simulink model "tanks_3_mathworks"  (Simulink 8.7)
settings: Solver=VariableStepAuto  StartTime=0.0  StopTime=700.0  RelTol=1e-3
values from neighbouring files (symbols this model uses):
  A1 = 4.9    [defineProcess_basic_outputs.m]
  g = 981    [defineProcess_basic_outputs.m]
  g1 = 0.3    [defineProcess_basic_outputs.m]
  g2 = 0.3    [defineProcess_basic_outputs.m]
  h1 = 10    [defineProcess_basic_outputs.m]
  h2 = 10    [defineProcess_basic_outputs.m]
  h3 = (k2*u2*(1-g2)/a3)^2/(2*g)    [defineProcess_basic_outputs.m]
  h4 = (k1*u1*(1-g1)/a4)^2/(2*g)    [defineProcess_basic_outputs.m]
  k1 = 1.6    [defineProcess_basic_outputs.m]
  k2 = 1.6    [defineProcess_basic_outputs.m]
  kc = [kc1 kc2 kc3 kc4]    [defineProcess_basic_outputs.m]
  kc1 = 0.5    [defineProcess_basic_outputs.m]
  kc2 = 0.5    [defineProcess_basic_outputs.m]
  kc3 = 0.5    [defineProcess_basic_outputs.m]
  kc4 = 0.5    [defineProcess_basic_outputs.m]
  Ts = 0.5    [defineProcess_basic_outputs.m]
  u1 = sqrt(2*g)*((g2-1)*a2*sqrt(h2)+g2*a1*sqrt(h1))/(k1*(g1+g2-1))    [defineProcess_basic_outputs.m]
  u2 = sqrt(2*g)*((g1-1)*a1*sqrt(h1)+g1*a2*sqrt(h2))/(k2*(g1+g2-1))    [defineProcess_basic_outputs.m]
undefined symbols (not defined in the file): a1, a2, A2, a3, A3, a4, A4
libraries: mpclib x1
settings Model: Creator=his10eni  LastModifiedBy=his10eni
settings DataIOCC: LimitDataPoints=off  SaveFormat=Dataset
settings DebuggingCC: UnderspecifiedInitializationDetection=Simplified  MergeDetectMultiDrivingBlocksExec=error
settings HardwareCC: ProdBitPerPointer=64  ProdLargestAtomicFloat=Float  ProdIntDivRoundTo=Zero  ProdEndianess=LittleEndian  ProdWordSize=64  ProdHWDeviceType=Intel->x86-64 (Windows64)
settings ModelReferenceCC: PropagateSignalLabelsOutOfModel=on
settings ConfigComp: CovModelRefEnable=off

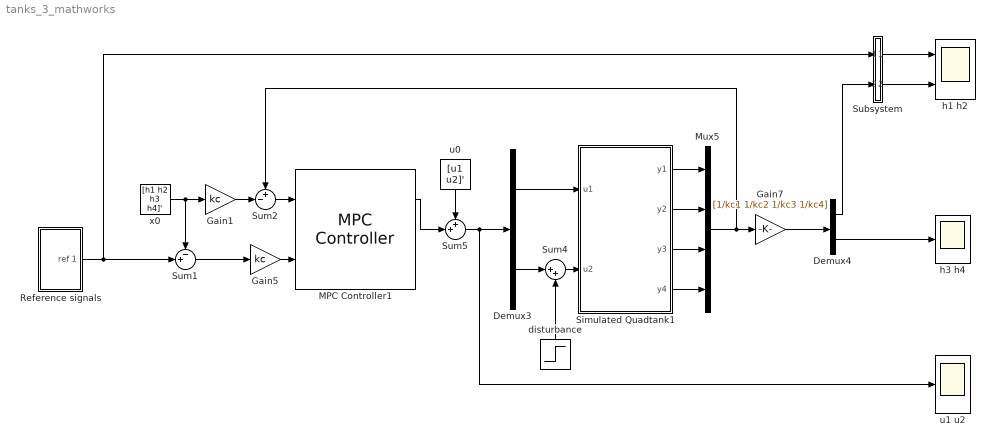
== system tanks_3_mathworks ==
  Demux3 : Demux  Outputs=2
  Demux4 : Demux  Outputs=2
  Gain1 : Gain  Gain=kc
  Gain5 : Gain  Gain=kc
  Gain7 : Gain  Gain=[1/kc1 1/kc2 1/kc3 1/kc4]
  MPC Controller1 : mpclib/MPC Controller  SCDEnableBlockLinearizationSpecification=on  mpcobj=mpcobj  is_multiple=0  enable_value=0  return_u0=off  ref_from_ws=off  ref_signal_name=[]  ref_preview=off  md_from_ws=off  md_signal_name=[]  md_preview=off  from_project=off  project_file=MPCtask.mat  md_inport=off  mv_inport=off  cost_outport=off  return_sequence=off  return_qpstatus=off  return_state=on  state_inport=off  lims_inport=off  ywt_inport=off  is_designfromscratch=0  uwt_inport=off  duwt_inport=off  rhoeps_inport=off  uref_inport=off  n_ts=0.5  n_mv=2  n_md=0  n_ud=0  n_mo=4  n_uo=0  BlockDataType=double  SampleTimeInherited=off  switch_inport=off
  Mux5 : Mux
  Reference signals : Subsystem
  Simulated Quadtank1 : Subsystem
  Subsystem : Subsystem
  Sum1 : Sum  Inputs=-+|  SaturateOnIntegerOverflow=on  InputSameDT=on  OutDataTypeStr=Inherit: Same as first input
  Sum2 : Sum  Inputs=+-|  SaturateOnIntegerOverflow=on  InputSameDT=on  OutDataTypeStr=Inherit: Same as first input
  Sum4 : Sum  Inputs=|++  SaturateOnIntegerOverflow=on  InputSameDT=on  OutDataTypeStr=Inherit: Same as first input
  Sum5 : Sum  Inputs=++|  SaturateOnIntegerOverflow=on  InputSameDT=on  OutDataTypeStr=Inherit: Same as first input
  disturbance : Step  Time=600  After=2  SampleTime=Ts
  h1 h2 : Scope  NumInputPorts=2
  h3 h4 : Scope
  u0 : Constant  Value=[u1 u2]'
  u1 u2 : Scope
  x0 : Constant  Value=[h1 h2 h3 h4]'
  wires:
  u0/1 -> Sum5/1
  Simulated Quadtank1/2(y2) -> Mux5/2
  Demux4/2 -> h3 h4/1
  Simulated Quadtank1/3(y3) -> Mux5/3
  Simulated Quadtank1/4(y4) -> Mux5/4
  Sum1/1 -> Gain5/1
  MPC Controller1/1 -> Sum5/2
  Sum2/1 -> MPC Controller1/1
  Gain5/1 -> MPC Controller1/2
  Demux3/1 -> Simulated Quadtank1/1(u1)
  Demux3/2 -> Sum4/1
  Sum4/1 -> Simulated Quadtank1/2(u2)
  disturbance/1 -> Sum4/2
  Mux5/1 -> Gain7/1, Sum2/1
  Subsystem/1(ref1 x1) -> h1 h2/1
  Subsystem/2(ref2 x2) -> h1 h2/2
  Demux4/1 -> Subsystem/2(x1 x2)
  Sum5/1 -> Demux3/1, u1 u2/1
  Reference signals/1(ref 1) -> Subsystem/1(reference signals), Sum1/2
  Simulated Quadtank1/1(y1) -> Mux5/1
  Gain7/1 -> Demux4/1
  Gain1/1 -> Sum2/2
  x0/1 -> Gain1/1, Sum1/1

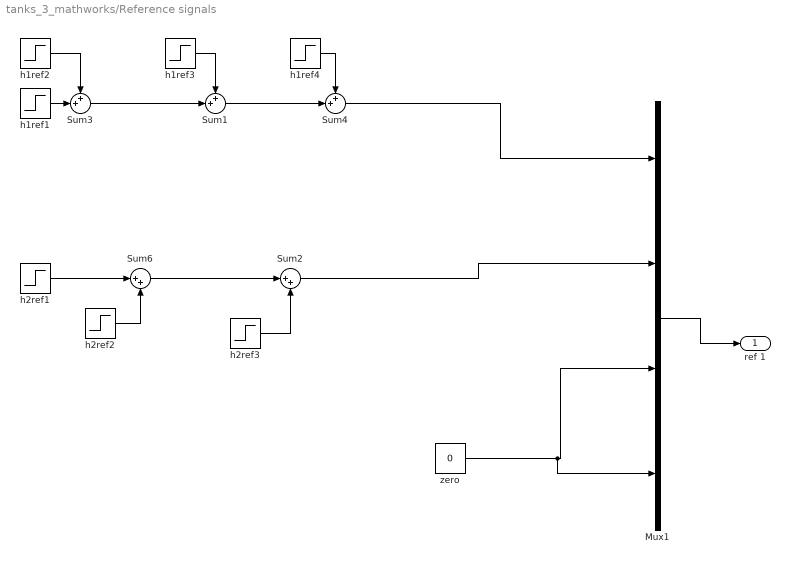
== system tanks_3_mathworks/Reference signals ==
  Mux1 : Mux
  Sum1 : Sum  Inputs=++|  SaturateOnIntegerOverflow=on  InputSameDT=on  OutDataTypeStr=Inherit: Same as first input
  Sum2 : Sum  Inputs=|++  SaturateOnIntegerOverflow=on  InputSameDT=on  OutDataTypeStr=Inherit: Same as first input
  Sum3 : Sum  Inputs=++|  SaturateOnIntegerOverflow=on  InputSameDT=on  OutDataTypeStr=Inherit: Same as first input
  Sum4 : Sum  Inputs=++|  SaturateOnIntegerOverflow=on  InputSameDT=on  OutDataTypeStr=Inherit: Same as first input
  Sum6 : Sum  Inputs=|++  SaturateOnIntegerOverflow=on  InputSameDT=on  OutDataTypeStr=Inherit: Same as first input
  h1ref1 : Step  Time=0  After=13  SampleTime=Ts
  h1ref2 : Step  Time=100  After=-5  SampleTime=Ts
  h1ref3 : Step  Time=300  After=4  SampleTime=Ts
  h1ref4 : Step  Time=500  After=-3  SampleTime=Ts
  h2ref1 : Step  Time=0  After=5  SampleTime=Ts
  h2ref2 : Step  Time=200  After=7  SampleTime=Ts  ZeroCross=off
  h2ref3 : Step  Time=400  After=-4  SampleTime=Ts  ZeroCross=off
  zero : Constant  Value=0  SampleTime=Ts
  ref 1 : Outport
  wires:
  h1ref4/1 -> Sum4/1
  Sum1/1 -> Sum4/2
  h2ref3/1 -> Sum2/2
  Sum6/1 -> Sum2/1
  h1ref3/1 -> Sum1/1
  Sum3/1 -> Sum1/2
  h2ref1/1 -> Sum6/1
  h1ref1/1 -> Sum3/2
  h2ref2/1 -> Sum6/2
  h1ref2/1 -> Sum3/1
  Mux1/1 -> ref 1/1
  Sum4/1 -> Mux1/1
  Sum2/1 -> Mux1/2
  zero/1 -> Mux1/4, Mux1/3

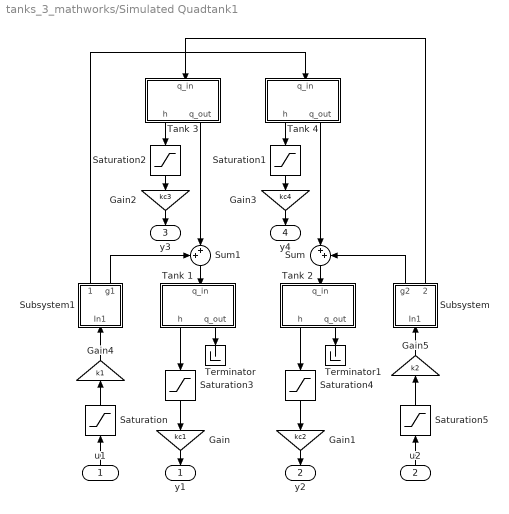
== system tanks_3_mathworks/Simulated Quadtank1 ==
  u1 : Inport
  u2 : Inport  Port=2
  Gain : Gain  Gain=kc1
  Gain1 : Gain  Gain=kc2
  Gain2 : Gain  Gain=kc3
  Gain3 : Gain  Gain=kc4
  Gain4 : Gain  Gain=k1
  Gain5 : Gain  Gain=k2
  Saturation : Saturate  UpperLimit=10  LowerLimit=0  LinearizeAsGain=off  ZeroCross=off
  Saturation{1..4} (4 alike) : Saturate  UpperLimit=16  LowerLimit=0  LinearizeAsGain=off  ZeroCross=off
  Saturation5 : Saturate  UpperLimit=10  LowerLimit=0  LinearizeAsGain=off  ZeroCross=off
  Subsystem : Subsystem
  Subsystem1 : Subsystem
  Sum : Sum  Inputs=|++
  Sum1 : Sum  Inputs=++|
  Tank 1 : Subsystem  mask{h0=eps, a=a1, A1=A1, g=g}
      mask prompts: h0 "h0 [cm]"; a "a [cm^2]"; A1 "A [cm^2]"; g "g [cm/s^2]"
  Tank 2 : Subsystem  mask{h0=eps, a=a2, A1=A2, g=g}
      mask prompts: h0 "h0 [cm]"; a "a [cm^2]"; A1 "A [cm^2]"; g "g [cm/s^2]"
  Tank 3 : Subsystem  mask{h0=eps, a=a3, A1=A3, g=g}
      mask prompts: h0 "h0 [cm]"; a "a [cm^2]"; A1 "A [cm^2]"; g "g [cm/s^2]"
  Tank 4 : Subsystem  mask{h0=eps, a=a4, A1=A4, g=g}
      mask prompts: h0 "h0 [cm]"; a "a [cm^2]"; A1 "A [cm^2]"; g "g [cm/s^2]"
  Terminator : Terminator
  Terminator1 : Terminator
  y1 : Outport
  y2 : Outport  Port=2
  y3 : Outport  Port=3
  y4 : Outport  Port=4
  wires:
  u1/1 -> Saturation/1
  Saturation/1 -> Gain4/1
  Saturation5/1 -> Gain5/1
  u2/1 -> Saturation5/1
  Tank 2/1(h) -> Saturation4/1
  Saturation4/1 -> Gain1/1
  Tank 1/1(h) -> Saturation3/1
  Saturation3/1 -> Gain/1
  Saturation1/1 -> Gain3/1
  Tank 4/1(h) -> Saturation1/1
  Saturation2/1 -> Gain2/1
  Tank 3/1(h) -> Saturation2/1
  Gain5/1 -> Subsystem/1(In1)
  Gain4/1 -> Subsystem1/1(In1)
  Subsystem1/1(1-g1) -> Tank 4/1(q_in)
  Subsystem/2(1-g2) -> Tank 3/1(q_in)
  Subsystem1/2(g1) -> Sum1/1
  Subsystem/1(g2) -> Sum/2
  Tank 3/2(q_out) -> Sum1/2
  Sum1/1 -> Tank 1/1(q_in)
  Tank 4/2(q_out) -> Sum/1
  Sum/1 -> Tank 2/1(q_in)
  Gain3/1 -> y4/1
  Gain2/1 -> y3/1
  Gain1/1 -> y2/1
  Tank 2/2(q_out) -> Terminator1/1
  Tank 1/2(q_out) -> Terminator/1
  Gain/1 -> y1/1

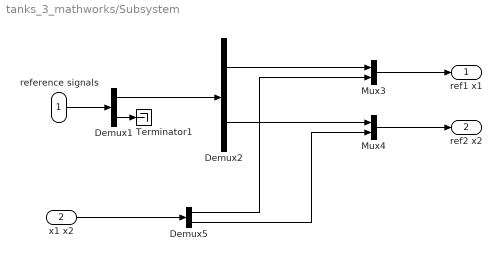
== system tanks_3_mathworks/Subsystem ==
  reference signals : Inport
  x1 x2 : Inport  Port=2
  Demux1 : Demux  Outputs=2
  Demux2 : Demux  Outputs=2
  Demux5 : Demux  Outputs=2
  Mux3 : Mux  Inputs=2
  Mux4 : Mux  Inputs=2
  Terminator1 : Terminator
  ref1 x1 : Outport
  ref2 x2 : Outport  Port=2
  wires:
  Demux2/1 -> Mux3/1
  Demux1/2 -> Terminator1/1
  Demux2/2 -> Mux4/1
  Demux5/1 -> Mux3/2
  Demux5/2 -> Mux4/2
  Demux1/1 -> Demux2/1
  reference signals/1 -> Demux1/1
  Mux4/1 -> ref2 x2/1
  Mux3/1 -> ref1 x1/1
  x1 x2/1 -> Demux5/1

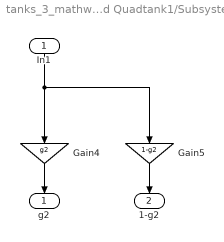
== system tanks_3_mathworks/Simulated Quadtank1/Subsystem ==
  In1 : Inport
  Gain4 : Gain  Gain=g2
  Gain5 : Gain  Gain=1-g2
  g2 : Outport
  1-g2 : Outport  Port=2
  wires:
  Gain5/1 -> 1-g2/1
  Gain4/1 -> g2/1
  In1/1 -> Gain4/1, Gain5/1

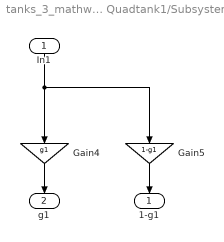
== system tanks_3_mathworks/Simulated Quadtank1/Subsystem1 ==
  In1 : Inport
  Gain4 : Gain  Gain=g1
  Gain5 : Gain  Gain=1-g1
  1-g1 : Outport
  g1 : Outport  Port=2
  wires:
  Gain4/1 -> g1/1
  Gain5/1 -> 1-g1/1
  In1/1 -> Gain4/1, Gain5/1

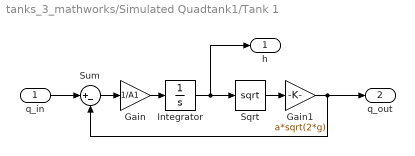
== system tanks_3_mathworks/Simulated Quadtank1/Tank 1 ==
  q_in : Inport
  Gain : Gain  Gain=1/A1
  Gain1 : Gain  Gain=a*sqrt(2*g)
  Integrator : Integrator  InitialCondition=h0  LimitOutput=on  UpperSaturationLimit=16  LowerSaturationLimit=eps
  Sqrt : Sqrt  SaturateOnIntegerOverflow=on
  Sum : Sum  Inputs=|+-
  h : Outport
  q_out : Outport  Port=2
  wires:
  q_in/1 -> Sum/1
  Sqrt/1 -> Gain1/1
  Gain1/1 -> Sum/2, q_out/1
  Sum/1 -> Gain/1
  Integrator/1 -> Sqrt/1, h/1
  Gain/1 -> Integrator/1

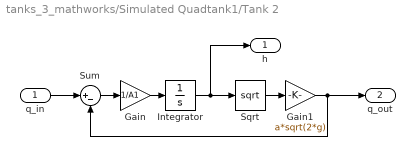
== system tanks_3_mathworks/Simulated Quadtank1/Tank 2 ==
  q_in : Inport
  Gain : Gain  Gain=1/A1
  Gain1 : Gain  Gain=a*sqrt(2*g)
  Integrator : Integrator  InitialCondition=h0  LimitOutput=on  UpperSaturationLimit=16  LowerSaturationLimit=eps
  Sqrt : Sqrt  SaturateOnIntegerOverflow=on
  Sum : Sum  Inputs=|+-
  h : Outport
  q_out : Outport  Port=2
  wires:
  q_in/1 -> Sum/1
  Sqrt/1 -> Gain1/1
  Gain1/1 -> Sum/2, q_out/1
  Sum/1 -> Gain/1
  Integrator/1 -> Sqrt/1, h/1
  Gain/1 -> Integrator/1

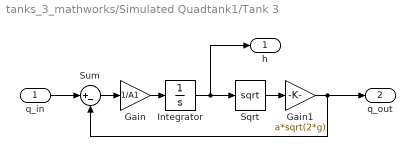
== system tanks_3_mathworks/Simulated Quadtank1/Tank 3 ==
  q_in : Inport
  Gain : Gain  Gain=1/A1
  Gain1 : Gain  Gain=a*sqrt(2*g)
  Integrator : Integrator  InitialCondition=h0  LimitOutput=on  UpperSaturationLimit=16  LowerSaturationLimit=eps
  Sqrt : Sqrt  SaturateOnIntegerOverflow=on
  Sum : Sum  Inputs=|+-
  h : Outport
  q_out : Outport  Port=2
  wires:
  q_in/1 -> Sum/1
  Sqrt/1 -> Gain1/1
  Gain1/1 -> Sum/2, q_out/1
  Sum/1 -> Gain/1
  Integrator/1 -> Sqrt/1, h/1
  Gain/1 -> Integrator/1

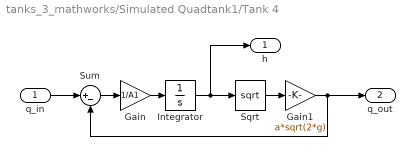
== system tanks_3_mathworks/Simulated Quadtank1/Tank 4 ==
  q_in : Inport
  Gain : Gain  Gain=1/A1
  Gain1 : Gain  Gain=a*sqrt(2*g)
  Integrator : Integrator  InitialCondition=h0  LimitOutput=on  UpperSaturationLimit=16  LowerSaturationLimit=eps
  Sqrt : Sqrt  SaturateOnIntegerOverflow=on
  Sum : Sum  Inputs=|+-
  h : Outport
  q_out : Outport  Port=2
  wires:
  q_in/1 -> Sum/1
  Sqrt/1 -> Gain1/1
  Gain1/1 -> Sum/2, q_out/1
  Sum/1 -> Gain/1
  Integrator/1 -> Sqrt/1, h/1
  Gain/1 -> Integrator/1
